simulink model "NeuralNetUnitLDC_IO"  (R2019a)
settings: Solver=FixedStepAuto  StartTime=0.0  StopTime=10  FixedStep=0.1  RelTol=1e-3
values from neighbouring files (symbols this model uses):
  B = 0.5    [System_parameters.m]
  b = f    (= 0.05)    [System_parameters.m]
  l = 0.6    [System_parameters.m]
  m = 0.250    (= 0.25)    [System_parameters.m]    (also in test1.m = 2)
  R = 0.1    [System_parameters.m]
settings Model: Creator=Therecia  LastModifiedBy=Tyson
settings DataIOCC: ReturnWorkspaceOutputs=off
settings DebuggingCC: InheritedTsInSrcMsg=none  PregeneratedLibrarySubsystemCodeDiagnostic=none  ArithmeticOperatorsInVariantConditions=warning
settings SFSimCC: SimUseLocalCustomCode=off
settings RTWCC: RTWUseLocalCustomCode=off
settings CodeAppCC: StateflowObjectComments=on

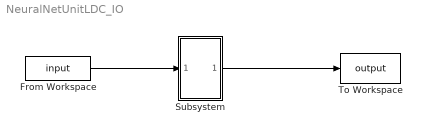
== system NeuralNetUnitLDC_IO ==
  From Workspace : FromWorkspace  VariableName=input
  Subsystem : Subsystem
      mask DialogControl Control2 Prompt: BlackBox
  To Workspace : ToWorkspace  VariableName=output  SaveFormat=Timeseries  SampleTime=-1
  wires:
  From Workspace/1 -> Subsystem/1(In1)
  Subsystem/1(Out1) -> To Workspace/1

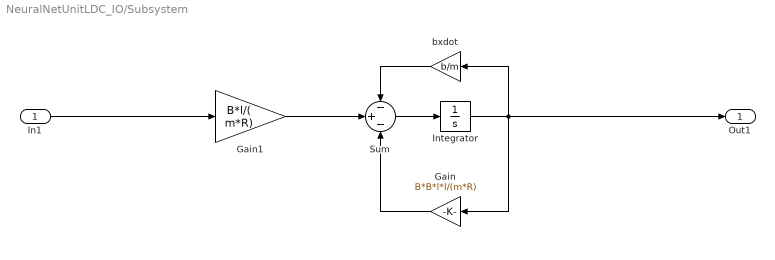
== system NeuralNetUnitLDC_IO/Subsystem ==
  In1 : Inport
  Gain : Gain  Gain=B*B*l*l/(m*R)
  Gain1 : Gain  Gain=B*l/( m*R)
  Integrator : Integrator
  Sum : Sum  Inputs=-+-
  bxdot : Gain  Gain=b/m
  Out1 : Outport
  wires:
  Sum/1 -> Integrator/1
  Gain/1 -> Sum/3
  Gain1/1 -> Sum/2
  bxdot/1 -> Sum/1
  Integrator/1 -> Out1/1, bxdot/1, Gain/1
  In1/1 -> Gain1/1
